simulink model "kidney2019"  (R2019a)
settings: Solver=VariableStepAuto  StartTime=0.0  StopTime=10000  RelTol=1e-3
undefined symbols (not defined in the file or in its folder): sigbuilder_block
settings Model: Creator=PUGAZH  LastModifiedBy=PUGAZH
settings DebuggingCC: SFMachineParentedDataDiag=error

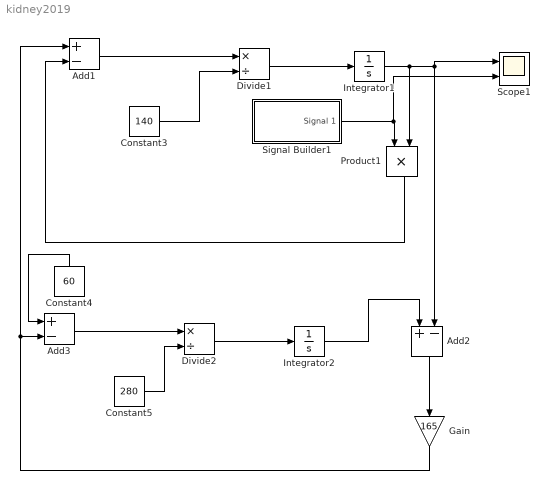
== system kidney2019 ==
  Add1 : Sum  Inputs=+-
  Add2 : Sum  Inputs=+-
  Add3 : Sum  Inputs=+-
  Constant3 : Constant  Value=140
  Constant4 : Constant  Value=60
  Constant5 : Constant  Value=280
  Divide1 : Product  Inputs=*/
  Divide2 : Product  Inputs=*/
  Gain : Gain  Gain=165
  Integrator1 : Integrator
  Integrator2 : Integrator
  Product1 : Product
  Scope1 : Scope  NumInputPorts=2
  Signal Builder1 : Subsystem  Tag=STV Subsys  LoadFcn=sigbuilder_block('load');  StartFcn=sigbuilder_block('start');  StopFcn=sigbuilder_block('stop');  ClipboardFcn=sigbuilder_block('clipboard');  mask(Sigbuilder block){tuvar=[0:10]}
      mask help: Simulink:masks:SigbuilderBlock_MD
      mask init:
      | if ~strcmp(get_param(bdroot(gcbh),'SimulationStatus'),'stopped') tuvar = sigbuilder_block('maskInit'); end
      settings: CopyFcn=sigbuilder_block('copy');  DeleteFcn=sigbuilder_block('delete');  ModelCloseFcn=sigbuilder_block('modelClose');  PreSaveFcn=sigbuilder_block('preSave');  PauseFcn=sigbuilder_block('pause');  ContinueFcn=sigbuilder_block('continue');  NameChangeFcn=sigbuilder_block('namechange');  OpenFcn=sigbuilder_block('open',[236.25 21 718.5 669 ]);  CloseFcn=sigbuilder_block('close');
      mask Display: plot(0, 0, 100, 100,[2, 2, 32, 32, 2], [68, 8, 8, 68, 68],[32, 2], [38, 38], [32, 19, 2],[53, 60, 44], [32, 17, 17, 2],[16, 16, 31, 31]);txt = getActiveGroup(gcbh);text(2, 100, txt,'verticalAlignment', 'top');
  wires:
  Product1/1 -> Add1/2
  Signal Builder1/1(Signal 1) -> Scope1/2, Product1/1
  Gain/1 -> Add3/2, Add1/1
  Constant3/1 -> Divide1/2
  Add1/1 -> Divide1/1
  Integrator1/1 -> Product1/2, Add2/2, Scope1/1
  Divide1/1 -> Integrator1/1
  Constant4/1 -> Add3/1
  Add3/1 -> Divide2/1
  Divide2/1 -> Integrator2/1
  Integrator2/1 -> Add2/1
  Constant5/1 -> Divide2/2
  Add2/1 -> Gain/1

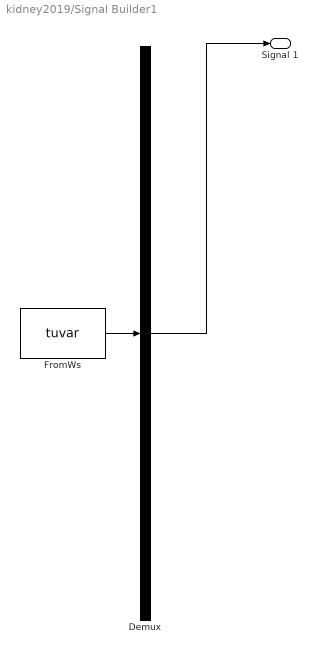
== system kidney2019/Signal Builder1 ==
  Demux : Demux  Tag=STV Demux  Outputs=1
      settings: DisplayOption=none
  FromWs : FromWorkspace  Tag=STV FromWs  VariableName=tuvar
      SigBuilderData=|
      | common.afterFinalStr = 'Extrapolate'
      | common.sampleTime = 0
      | dataSet.timeRange = [0 10000]
      | dataSet.name = 'Group 1'
      | sbobj.Groups.Name = 'Group 1'
      | sbobj.Groups.Signals.Name = 'Signal 1'
      | sbobj.Groups.Signals.XData = [0 1000 2000 3000 4000 5000 6000 7000 8000 9000 10000]
      | sbobj.Groups.Signals.YData = [0 0 10 20 150 500 400 300 150 50 0]
      | sbobj.Groups.TimeRange = [0 10000]
  Signal 1 : Outport  Tag=STV Outport
  wires:
  FromWs/1 -> Demux/1
  Demux/1 -> Signal 1/1
